simulink model "conv_exp_func"  (R2016a)
settings: Solver=VariableStepAuto  StartTime=0.0  StopTime=10.0  RelTol=1e-3
libraries: dspsrcs4 x2, dspsigops x1
settings Model: Creator=Chris  LastModifiedBy=Chris

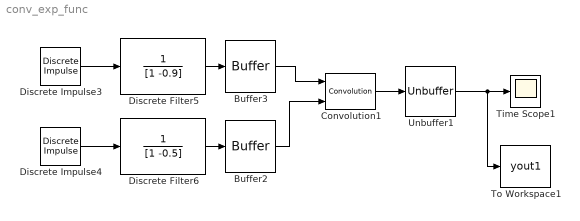
== system conv_exp_func ==
  Buffer2 : Buffer  N=50  TreatMby1Signals=One channel
  Buffer3 : Buffer  N=50  TreatMby1Signals=One channel
  Convolution1 : dspsigops/Convolution  domain=Time  outputDataTypeStr=Inherit: Same as accumulator  outputLastDataTypeStr=Inherit: Same as accumulator  outputMin=[]  outputMax=[]  roundingMode=Floor  overflowMode=off
  Discrete Impulse3 : dspsrcs4/Discrete  Impulse  Delay=0  SampleTime=1  FrameSample=1  OutputFrames=on  dataType=double  isSigned=on  wordLen=16  udDataType=sfix(16)  fracBitsMode=Best precision  numFracBits=15  OutDataTypeStr=double  LastOutDataTypeStr=double
  Discrete Impulse4 : dspsrcs4/Discrete  Impulse  Delay=0  SampleTime=1  FrameSample=1  OutputFrames=on  dataType=double  isSigned=on  wordLen=16  udDataType=sfix(16)  fracBitsMode=Best precision  numFracBits=15  OutDataTypeStr=double  LastOutDataTypeStr=double
  Discrete Filter5 : DiscreteFilter  Numerator=1  Denominator=[1 -0.9]  InputProcessing=Columns as channels (frame based)  FilterStructure=Direct form II transposed  a0EqualsOne=on
  Discrete Filter6 : DiscreteFilter  Numerator=1  Denominator=[1 -0.5]  InputProcessing=Columns as channels (frame based)  FilterStructure=Direct form II transposed  a0EqualsOne=on
  Time Scope1 : Scope
  To Workspace1 : ToWorkspace  VariableName=yout1  SampleTime=-1
      settings: Save2DSignal=2-D array (concatenate along first dimension)
  Unbuffer1 : Unbuffer  SampleBasedProcessing=Same as frame based
  wires:
  Buffer2/1 -> Convolution1/2
  Unbuffer1/1 -> To Workspace1/1, Time Scope1/1
  Discrete Filter5/1 -> Buffer3/1
  Buffer3/1 -> Convolution1/1
  Convolution1/1 -> Unbuffer1/1
  Discrete Filter6/1 -> Buffer2/1
  Discrete Impulse3/1 -> Discrete Filter5/1
  Discrete Impulse4/1 -> Discrete Filter6/1
